simulink model "SimulinkLinear1"  (Simulink 8.2)
settings: Solver=ode5  StartTime=0.0  StopTime=20  FixedStep=0.01  RelTol=1e-3
undefined symbols (not defined in the file or in its folder): A_Lat, A_Long, B_Lat, B_Long, C_Lat, C_Long, D_Lat, D_Long, sigbuilder_block
libraries: simulink_extras x2
settings Model: Creator=AGSilva  LastModifiedBy=AGSilva
settings DataIOCC: SaveFormat=StructureWithTime  SignalLoggingSaveFormat=Dataset  SaveOutput=off  SaveTime=off
settings OptimizationCC: InitFltsAndDblsToZero=on
settings DebuggingCC: SaveWithParameterizedLinksMsg=none
settings GRTTargetCC: TargetFcnLib=ansi_tfl_tmw.mat

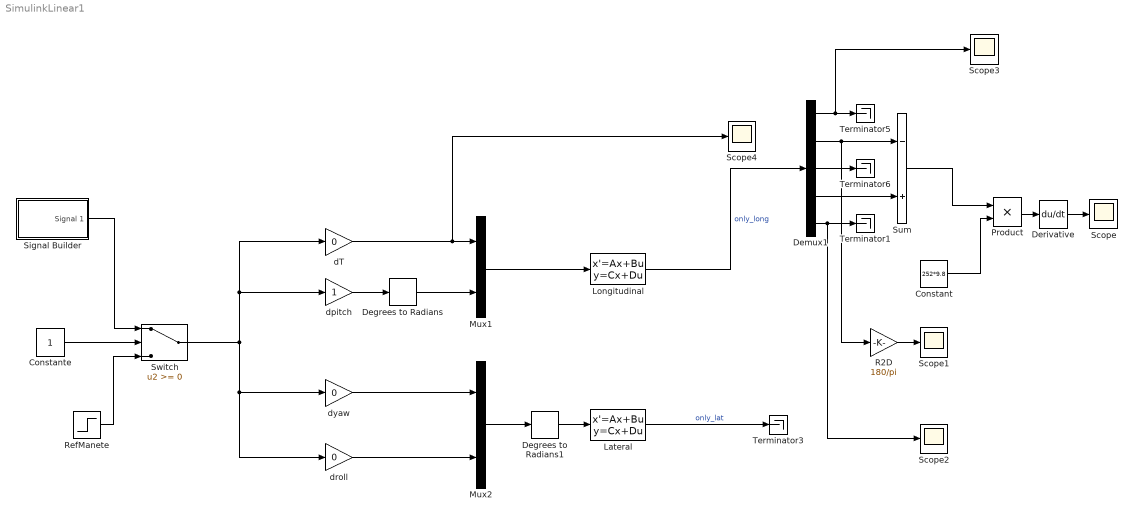
== system SimulinkLinear1 ==
  Constant : Constant  Value=252*9.8
  Constante : Constant
  Degrees to Radians : simulink_extras/Transformations/Degrees to Radians
  Degrees to Radians1 : simulink_extras/Transformations/Degrees to Radians
  Demux1 : Demux  Outputs=5
  Derivative : Derivative
  Lateral : StateSpace  A=A_Lat  B=B_Lat  C=C_Lat  D=D_Lat  X0=0
  Longitudinal : StateSpace  A=A_Long  B=B_Long  C=C_Long  D=D_Long  X0=0
  Mux1 : Mux  Inputs=2
  Mux2 : Mux  Inputs=2
  Product : Product
  R2D : Gain  Gain=180/pi
  RefManete : Step  After=0.05  SampleTime=0  VectorParams1D=off
  Scope{,1..4} (5 alike) : Scope
      Scope2 settings: SaveName=ScopeData2
      Scope3 settings: SaveName=ScopeData3
      Scope4 settings: SaveName=ScopeData4
  Signal Builder : Subsystem  Tag=STV Subsys  LoadFcn=sigbuilder_block('load');  StartFcn=sigbuilder_block('start');  StopFcn=sigbuilder_block('stop');  ClipboardFcn=sigbuilder_block('clipboard');  mask(Sigbuilder block){}
      mask help: Sigbuilder GUI
      mask init:
      | if ~strcmp(get_param(bdroot(gcbh),'SimulationStatus'),'stopped') tuvar = sigbuilder_block('maskInit'); end
      settings: CopyFcn=sigbuilder_block('copy');  DeleteFcn=sigbuilder_block('delete');  ModelCloseFcn=sigbuilder_block('modelClose');  PreSaveFcn=sigbuilder_block('preSave');  PauseFcn=sigbuilder_block('pause')  ContinueFcn=sigbuilder_block('continue')  NameChangeFcn=sigbuilder_block('namechange');  OpenFcn=sigbuilder_block('open',[6 28.5 1248 693 ]);  CloseFcn=sigbuilder_block('close');
      mask Display: plot(0,0,100,100,[10,10,40,40,10],[80,20,20,80,80],[40,10],[50,50], [40,27,10],[65,72,56],[40,25,25,10],[28,28,43,43]);
  Sum : Sum  Inputs=-+
  Switch : Switch
  Terminator{1,3,5..6} (4 alike) : Terminator
  dT : Gain  Gain=0
  dpitch : Gain
  droll : Gain  Gain=0
  dyaw : Gain  Gain=0
  wires:
  dpitch/1 -> Degrees to Radians/1
  dyaw/1 -> Mux2/1
  droll/1 -> Mux2/2
  Longitudinal/1 -> Demux1/1  "only_long"
  Mux1/1 -> Longitudinal/1
  Mux2/1 -> Degrees to Radians1/1
  Lateral/1 -> Terminator3/1  "only_lat"
  Demux1/2 -> R2D/1, Sum/1
  Constant/1 -> Product/2
  Product/1 -> Derivative/1
  Derivative/1 -> Scope/1
  RefManete/1 -> Switch/3
  Sum/1 -> Product/1
  Demux1/4 -> Sum/2
  Demux1/1 -> Scope3/1, Terminator5/1
  Demux1/3 -> Terminator6/1
  Signal Builder/1(Signal 1) -> Switch/1
  Switch/1 -> droll/1, dyaw/1, dpitch/1, dT/1
  Constante/1 -> Switch/2
  Demux1/5 -> Scope2/1, Terminator1/1
  dT/1 -> Scope4/1, Mux1/1
  R2D/1 -> Scope1/1
  Degrees to Radians/1 -> Mux1/2
  Degrees to Radians1/1 -> Lateral/1

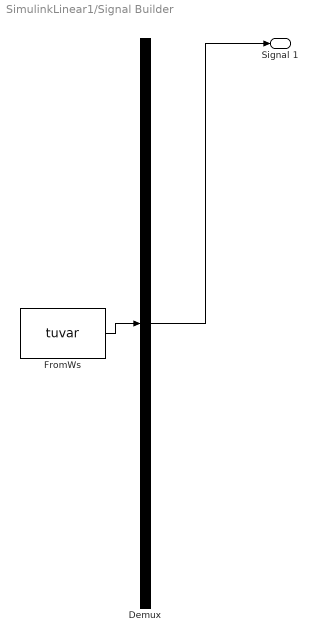
== system SimulinkLinear1/Signal Builder ==
  Demux : Demux  Tag=STV Demux  Outputs=1
  FromWs : FromWorkspace  Tag=STV FromWs  VariableName=tuvar  SampleTime=0  SigBuilderData=DataTag0  VnvData=DataTag1
      SigBuilderData=|
      | common.afterFinalStr = 'Extrapolate'
      | common.sampleTime = 0
      | dataSet.timeRange = [0 10]
      | dataSet.name = 'Group 1'
      | sbobj.Groups.Name = 'Group 1'
      | sbobj.Groups.Signals.Name = 'Signal 1'
      | sbobj.Groups.Signals.XData = [0 1 1 1.25 1.25 1.5 1.5 10]
      | sbobj.Groups.Signals.YData = [0 0 1 1 -1 -1 0 0]
  Signal 1 : Outport  Tag=STV Outport
  wires:
  Demux/1 -> Signal 1/1
  FromWs/1 -> Demux/1
